simulink model "PID_explicit"  (R2016b)
settings: Solver=VariableStepAuto  StartTime=0.0  StopTime=10.0  RelTol=1e-3
undefined symbols (not defined in the file): kd, ki, kp
settings Model: Creator=bw_  LastModifiedBy=bw_

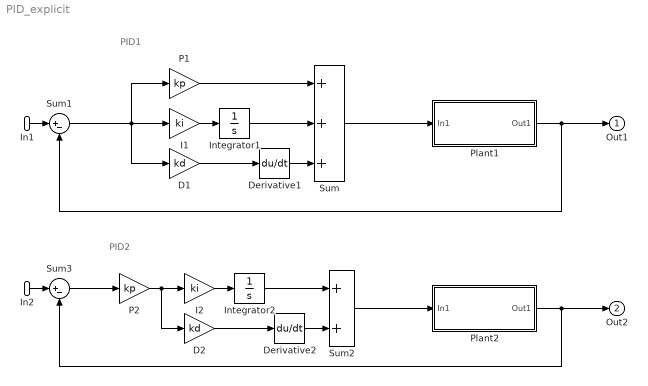
== system PID_explicit ==
  note: PID2
  note: PID1
  In1 : Inport
  In2 : Inport  Port=2
  D1 : Gain  Gain=kd
  D2 : Gain  Gain=kd
  Derivative1 : Derivative
  Derivative2 : Derivative
  I1 : Gain  Gain=ki
  I2 : Gain  Gain=ki
  Integrator1 : Integrator
  Integrator2 : Integrator
  P1 : Gain  Gain=kp
  P2 : Gain  Gain=kp
  Plant1 : Subsystem
  Plant2 : Subsystem
  Sum : Sum  Inputs=+++
  Sum1 : Sum  Inputs=|+-
  Sum2 : Sum
  Sum3 : Sum  Inputs=|+-
  Out1 : Outport
  Out2 : Outport  Port=2
  wires:
  Plant1/1(Out1) -> Sum1/2, Out1/1
  In1/1 -> Sum1/1
  Plant2/1(Out1) -> Sum3/2, Out2/1
  In2/1 -> Sum3/1
  Sum/1 -> Plant1/1(In1)
  Sum1/1 -> D1/1, P1/1, I1/1
  Derivative1/1 -> Sum/3
  P1/1 -> Sum/1
  Integrator1/1 -> Sum/2
  D1/1 -> Derivative1/1
  I1/1 -> Integrator1/1
  Sum2/1 -> Plant2/1(In1)
  P2/1 -> D2/1, I2/1
  Sum3/1 -> P2/1
  Derivative2/1 -> Sum2/2
  I2/1 -> Integrator2/1
  Integrator2/1 -> Sum2/1
  D2/1 -> Derivative2/1

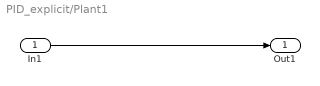
== system PID_explicit/Plant1 ==
  In1 : Inport
  Out1 : Outport
  wires:
  In1/1 -> Out1/1

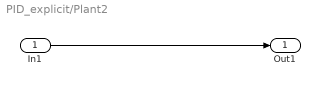
== system PID_explicit/Plant2 ==
  In1 : Inport
  Out1 : Outport
  wires:
  In1/1 -> Out1/1
